simulink model "M2"  (R2015b)
settings: Solver=VariableStepAuto  StartTime=-10  StopTime=10.0  RelTol=1e-3
libraries: simulink x1
settings Model: Creator=Pouya  LastModifiedBy=Pouya

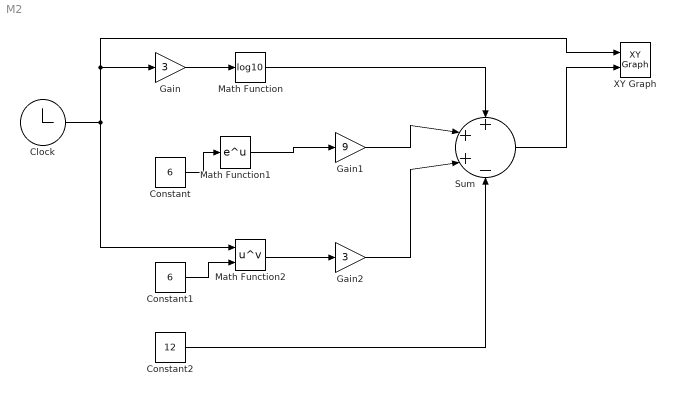
== system M2 ==
  Clock : Clock
  Constant : Constant  Value=6
  Constant1 : Constant  Value=6
  Constant2 : Constant  Value=12
  Gain : Gain  Gain=3
  Gain1 : Gain  Gain=9
  Gain2 : Gain  Gain=3
  Math Function : Math  Operator=log10  SaturateOnIntegerOverflow=on
  Math Function1 : Math  SaturateOnIntegerOverflow=on
  Math Function2 : Math  Operator=pow  SaturateOnIntegerOverflow=on
  Sum : Sum  Inputs=+++-
  XY Graph : simulink/Sinks/XY Graph  xmin=-100  xmax=100  ymin=-100  ymax=100  st=-1
  wires:
  Gain/1 -> Math Function/1
  Clock/1 -> XY Graph/1, Gain/1, Math Function2/1
  Constant/1 -> Math Function1/1
  Math Function1/1 -> Gain1/1
  Constant1/1 -> Math Function2/2
  Math Function2/1 -> Gain2/1
  Math Function/1 -> Sum/1
  Gain1/1 -> Sum/2
  Gain2/1 -> Sum/3
  Constant2/1 -> Sum/4
  Sum/1 -> XY Graph/2
